simulink model "aung"  (Simulink 5.0)
settings: Solver=ode45  StartTime=0.0  StopTime=1  RelTol=1e-3
libraries: simulink x8
settings Model: LastModifiedBy=Blue Phoenix  RTWOptions="-aEnforceIntegerDowncast=1 -aExtMode=0 -aExtModeTesting=0 -aFoldNonRolledExpr=1 -aForceParamTrailComments=0 -aGenerateComments=1 -aGenerateReport=0 -aIgnoreCustomStorageClasses=1 -aIncDataTypeInIds=0 -aIncHierarchyInIds=0 -aInlineInvariantSignals=0 -aInlinedPrmAccess=\"Literals\" -aLocalBlockOutputs=1 -aLogVarNameModifier=\"rt_\" -aMaxRTWIdLen=31 -aPrefixModelToSubsysFcnNames=1 -aRTWVerbose=1 -aRollThreshold=5 -aShowEliminatedStatements=0"

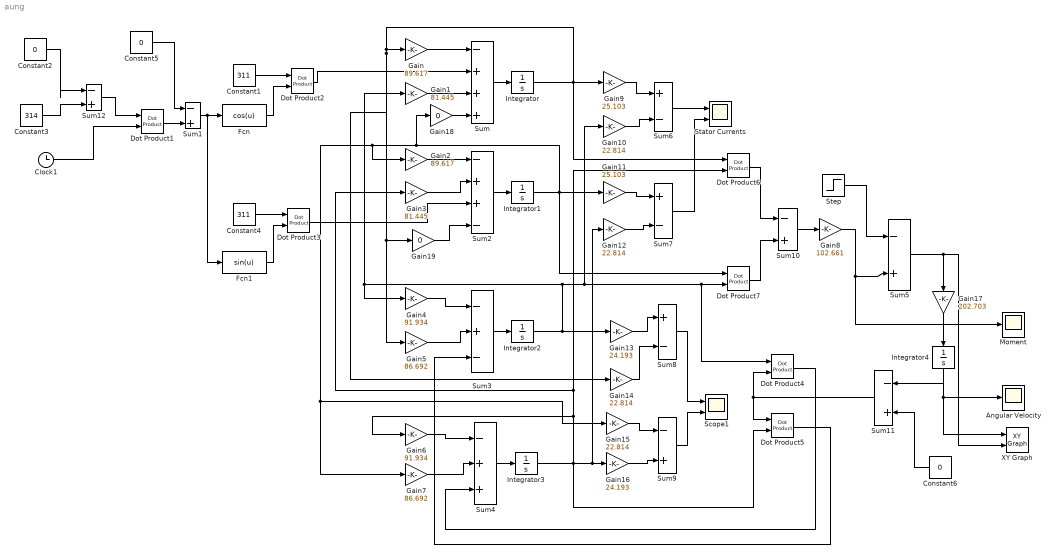
== system aung ==
  Angular Velocity : Scope
      settings: TimeRange=1  YMin=-3  YMax=8  SaveName=ScopeData4  SampleInput=on
  Clock1 : Clock
      settings: Decimation=10
  Constant1 : Constant  Value=311  ShowAdditionalParam=on
  Constant2 : Constant  Value=0  ShowAdditionalParam=on
  Constant3 : Constant  Value=314  ShowAdditionalParam=on
  Constant4 : Constant  Value=311  ShowAdditionalParam=on
  Constant5 : Constant  Value=0  ShowAdditionalParam=on
  Constant6 : Constant  Orientation=left  Value=0  ShowAdditionalParam=on
  Dot Product{1..7} (7 alike) : simulink/Math Operations/Dot Product
  Fcn : Fcn  Expr=cos(u)
  Fcn1 : Fcn  Expr=sin(u)
  Gain : Gain  Gain=89.617  ShowAdditionalParam=on  SaturateOnIntegerOverflow=on
  Gain1 : Gain  Gain=81.445  SaturateOnIntegerOverflow=on
  Gain{10,12,14..15} (4 alike) : Gain  Gain=22.814  SaturateOnIntegerOverflow=on
  Gain11 : Gain  Gain=25.103  SaturateOnIntegerOverflow=on
  Gain13 : Gain  Gain=24.193  SaturateOnIntegerOverflow=on
  Gain16 : Gain  Gain=24.193  SaturateOnIntegerOverflow=on
  Gain17 : Gain  Orientation=down  Gain=202.703  ShowAdditionalParam=on  SaturateOnIntegerOverflow=on
  Gain18 : Gain  Gain=0  SaturateOnIntegerOverflow=on
  Gain19 : Gain  Gain=0  SaturateOnIntegerOverflow=on
  Gain2 : Gain  Gain=89.617  SaturateOnIntegerOverflow=on
  Gain3 : Gain  Gain=81.445  SaturateOnIntegerOverflow=on
  Gain4 : Gain  Gain=91.934  SaturateOnIntegerOverflow=on
  Gain5 : Gain  Gain=86.692  SaturateOnIntegerOverflow=on
  Gain6 : Gain  Gain=91.934  SaturateOnIntegerOverflow=on
  Gain7 : Gain  Gain=86.692  SaturateOnIntegerOverflow=on
  Gain8 : Gain  Gain=102.661  SaturateOnIntegerOverflow=on
  Gain9 : Gain  Gain=25.103  SaturateOnIntegerOverflow=on
  Integrator{,1..3} (4 alike) : Integrator
  Integrator4 : Integrator  Orientation=down
  Moment : Scope
      settings: TimeRange=2  YMin=-2  YMax=8  SaveName=ScopeData2  SampleInput=on
  Scope1 : Scope  NumInputPorts=2
      settings: TimeRange=2  YMin=-20~-20  YMax=20~20
  Stator Currents : Scope  NumInputPorts=2
      settings: TimeRange=1  YMin=-20~-5  YMax=20~5  SampleInput=on
  Step : Step  Time=0  After=0  SampleTime=0
  Sum : Sum  Inputs=-+++  ShowAdditionalParam=on  SaturateOnIntegerOverflow=on
  Sum1 : Sum  Inputs=|-+  ShowAdditionalParam=on  SaturateOnIntegerOverflow=on
  Sum10 : Sum  Inputs=-+  ShowAdditionalParam=on  SaturateOnIntegerOverflow=on
  Sum11 : Sum  Orientation=left  Inputs=-+  ShowAdditionalParam=on  SaturateOnIntegerOverflow=on
  Sum12 : Sum  Inputs=|-+  ShowAdditionalParam=on  SaturateOnIntegerOverflow=on
  Sum2 : Sum  Inputs=-++-  ShowAdditionalParam=on  SaturateOnIntegerOverflow=on
  Sum3 : Sum  Inputs=-+-  ShowAdditionalParam=on  SaturateOnIntegerOverflow=on
  Sum4 : Sum  Inputs=-++  ShowAdditionalParam=on  SaturateOnIntegerOverflow=on
  Sum5 : Sum  Inputs=-+  ShowAdditionalParam=on  SaturateOnIntegerOverflow=on
  Sum6 : Sum  Inputs=+-  ShowAdditionalParam=on  SaturateOnIntegerOverflow=on
  Sum7 : Sum  Inputs=+-  ShowAdditionalParam=on  SaturateOnIntegerOverflow=on
  Sum8 : Sum  Inputs=+-  ShowAdditionalParam=on  SaturateOnIntegerOverflow=on
  Sum9 : Sum  Inputs=-+  ShowAdditionalParam=on  SaturateOnIntegerOverflow=on
  XY Graph : simulink/Sinks/XY Graph  xmin=-10  xmax=350  ymin=-3  ymax=8  st=-1
  wires:
  Sum1/1 -> Fcn/1, Fcn1/1
  Constant1/1 -> Dot Product2/1
  Dot Product1/1 -> Sum1/2
  Fcn1/1 -> Dot Product3/2
  Constant4/1 -> Dot Product3/1
  Sum4/1 -> Integrator3/1
  Sum3/1 -> Integrator2/1
  Sum2/1 -> Integrator1/1
  Sum/1 -> Integrator/1
  Integrator1/1 -> Dot Product7/1, Gain11/1, Gain2/1, Gain7/1, Gain15/1, Gain18/1
  Integrator2/1 -> Gain1/1, Gain4/1, Dot Product7/2, Dot Product4/1, Gain10/1, Gain13/1
  Integrator/1 -> Dot Product6/1, Gain9/1, Gain14/1, Gain5/1, Gain19/1, Gain/1
  Integrator3/1 -> Dot Product6/2, Gain3/1, Gain6/1, Dot Product5/2, Gain16/1, Gain12/1
  Dot Product6/1 -> Sum10/1
  Dot Product7/1 -> Sum10/2
  Sum10/1 -> Gain8/1
  Sum6/1 -> Stator Currents/1
  Sum8/1 -> Scope1/1
  Sum9/1 -> Scope1/2
  Step/1 -> Sum5/1
  Gain8/1 -> Sum5/2, Moment/1
  Gain17/1 -> Integrator4/1
  Sum5/1 -> Gain17/1, XY Graph/2
  Integrator4/1 -> XY Graph/1, Angular Velocity/1, Sum11/1
  Gain/1 -> Sum/1
  Gain4/1 -> Sum3/1
  Gain2/1 -> Sum2/1
  Fcn/1 -> Dot Product2/2
  Gain1/1 -> Sum/3
  Dot Product3/1 -> Sum2/3
  Gain6/1 -> Sum4/1
  Gain7/1 -> Sum4/2
  Gain5/1 -> Sum3/2
  Gain9/1 -> Sum6/1
  Gain10/1 -> Sum6/2
  Gain11/1 -> Sum7/1
  Gain12/1 -> Sum7/2
  Gain13/1 -> Sum8/1
  Gain14/1 -> Sum8/2
  Gain16/1 -> Sum9/2
  Gain15/1 -> Sum9/1
  Dot Product2/1 -> Sum/2
  Gain3/1 -> Sum2/2
  Sum7/1 -> Stator Currents/2
  Constant2/1 -> Sum12/1
  Constant3/1 -> Sum12/2
  Sum12/1 -> Dot Product1/1
  Clock1/1 -> Dot Product1/2
  Constant5/1 -> Sum1/1
  Gain18/1 -> Sum/4
  Gain19/1 -> Sum2/4
  Constant6/1 -> Sum11/2
  Sum11/1 -> Dot Product4/2, Dot Product5/1
  Dot Product4/1 -> Sum4/3
  Dot Product5/1 -> Sum3/3
